simulink model "flyback_converter_2"  (R2018a)
settings: Solver=VariableStepAuto  StartTime=0.0  StopTime=0.01  MaxStep=1e-6  RelTol=1e-3
libraries: powerlib x16
settings Model: Creator=FAHRİ TÜREDİ  LastModifiedBy=DELL

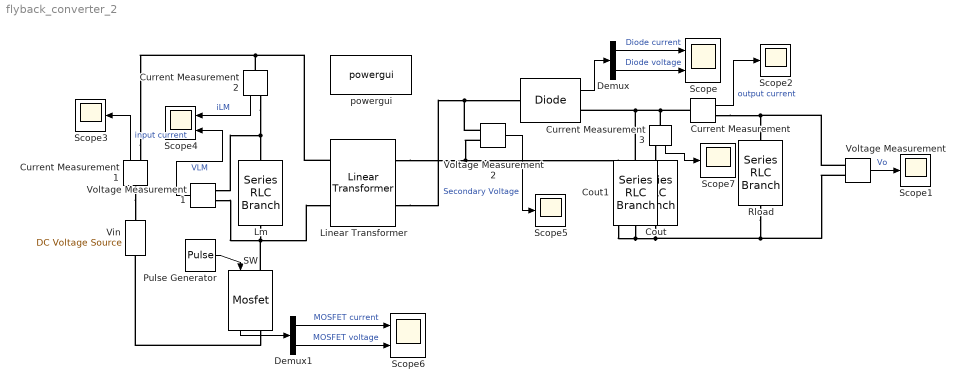
== system flyback_converter_2 ==
  Cout : powerlib/Elements/Series RLC Branch  LConnTagsString=__new0  RConnTagsString=__new0  BranchType=RC  Resistance=0.041  Inductance=28.67e-6  SetiL0=off  InitialCurrent=0  Capacitance=470e-6  Setx0=off  InitialVoltage=0  Measurements=None
  Cout1 : powerlib/Elements/Series RLC Branch  LConnTagsString=__new0  RConnTagsString=__new0  BranchType=RC  Resistance=0.041  Inductance=28.67e-6  SetiL0=off  InitialCurrent=0  Capacitance=470e-6  Setx0=off  InitialVoltage=0  Measurements=None
  Current Measurement{,1..3} (4 alike) : powerlib/Measurements/Current Measurement  PhasorSimulation=off  OutputType=Complex  PSBequivalent=0
  D : powerlib/Power Electronics/Diode  Ron=0.001  Lon=0  Vf=0  IC=0  UseSnubber=0  Rs=500  Cs=250e-9  Measurements=on
  Demux : Demux  Outputs=2
  Demux1 : Demux  Outputs=2
  Linear Transformer : powerlib/Elements/Linear Transformer  UNITS=SI  NominalPower=[ 100 45000 ]  winding1=[200 0 0]  winding2=[105.263 0 0]  ThreeWindings=off  winding3=[3.15e+05 0.7938 0.084225]  RmLm=[1.0805e+06 inf]  Measurements=None  DataType=on
  Lm : powerlib/Elements/Series RLC Branch  LConnTagsString=__new0  RConnTagsString=__new0  BranchType=L  Resistance=1  Inductance=28.67e-6  SetiL0=off  InitialCurrent=0  Capacitance=1e-6  Setx0=off  InitialVoltage=0  Measurements=None
  Pulse Generator : DiscretePulseGenerator  PulseType=Time based  Amplitude=5  Period=1/(45000)  PulseWidth=52
  Rload : powerlib/Elements/Series RLC Branch  LConnTagsString=__new0  RConnTagsString=__new0  BranchType=R  Resistance=15/4  Inductance=28.67e-6  SetiL0=off  InitialCurrent=0  Capacitance=1e-6  Setx0=off  InitialVoltage=0  Measurements=None
  SW : powerlib/Power Electronics/Mosfet  Ron=0.1  Lon=0  Rd=0.01  Vfd=0  IC=0  Rs=1e5  Cs=inf  Measurements=on
  Scope : Scope  NumInputPorts=2
  Scope{1..3,5,7} (5 alike) : Scope
  Scope4 : Scope  NumInputPorts=2
  Scope6 : Scope  NumInputPorts=2
  Vin : powerlib/Electrical Sources/DC Voltage Source  Amplitude=24  Measurements=None
  Voltage Measurement : powerlib/Measurements/Voltage Measurement  PhasorSimulation=off  OutputType=Complex  PSBequivalent=0
  Voltage Measurement1 : powerlib/Measurements/Voltage Measurement  PhasorSimulation=off  OutputType=Complex  PSBequivalent=0
  Voltage Measurement2 : powerlib/Measurements/Voltage Measurement  PhasorSimulation=off  OutputType=Complex  PSBequivalent=0
  powergui : powerlib/powergui  Priority=1  SimulationMode=Continuous  SampleTime=50e-6  frequency=60  Iterations=50  frequencyindice=0  Pbase=100e6  ErrMax=1e-4  UnitsV=kV  UnitsW=MW  buscounter=0  FunctionMessages=off  echomessages=off  EnableUseOfTLC=off  CurrentSourceSwitches=off  DisableSnubberDevices=off  DisableRonSwitches=off  DisableVfSwitches=off  DisplayEquations=off  SolverType=Tustin/Backward Euler (TBE)  Interpol=off  ExternalGateDelay=off  methode=off  Ts=100  x0status=blocks  SPID=on  SwTol=0  HookPort=off  RestoreLinks=warning  ResistiveCurrentMeasurement=off  Frange=[0:2:500]  Ylog=off  Xlog=on  ShowGrid=off  save=off  variable=ZData  structure=0  ZoomFFT=off  StartTime=0.0  cycles=1  DisplayStyle=1  fundamental=60  FreqAxis=off  MaxFrequency=1000  frequencyindicesteady=1  RmsSteady=1  display=off
  wires:
  Pulse Generator/1 -> SW/1
  Demux/1 -> Scope/1  "Diode current"
  Demux/2 -> Scope/2  "Diode voltage"
  D/1 -> Demux/1
  Voltage Measurement/1 -> Scope1/1  "Vo"
  Current Measurement/1 -> Scope2/1  "output current"
  Current Measurement1/1 -> Scope3/1  "input current"
  Current Measurement2/1 -> Scope4/1  "iLM"
  Voltage Measurement1/1 -> Scope4/2  "VLM"
  Demux1/1 -> Scope6/1  "MOSFET current"
  Demux1/2 -> Scope6/2  "MOSFET voltage"
  SW/1 -> Demux1/1
  Voltage Measurement2/1 -> Scope5/1  "Secondary Voltage"
  Current Measurement3/1 -> Scope7/1
  connections:
  Lm/RConn1 -- Linear Transformer/LConn2 -- Voltage Measurement1/LConn2 -- SW/LConn1
  SW/RConn1 -- Vin/LConn1
  Voltage Measurement2/LConn2 -- Linear Transformer/RConn2 -- D/LConn1
  Current Measurement/LConn1 -- Cout1/LConn1 -- D/RConn1 -- Current Measurement3/LConn1
  Cout/RConn1 -- Voltage Measurement2/LConn1 -- Linear Transformer/RConn1 -- Cout1/RConn1 -- Voltage Measurement/LConn2 -- Rload/RConn1
  Voltage Measurement/LConn1 -- Current Measurement/RConn1 -- Rload/LConn1
  Current Measurement1/LConn1 -- Vin/RConn1
  Current Measurement1/RConn1 -- Linear Transformer/LConn1 -- Current Measurement2/LConn1
  Current Measurement2/RConn1 -- Voltage Measurement1/LConn1 -- Lm/LConn1
  Current Measurement3/RConn1 -- Cout/LConn1
